simulink model "Simulation"  (R2020b)
settings: Solver=VariableStepAuto  StartTime=0.0  StopTime=10  RelTol=1e-3
model workspace (MAT data in the model file):
  DGain = Simulink.Parameter
  DGain.DataType = 'auto'
  DGain.Dimensions = [0 0]
  IGain = Simulink.Parameter
  IGain.DataType = 'auto'
  IGain.Dimensions = [0 0]
  PGain = Simulink.Parameter
  PGain.DataType = 'auto'
  PGain.Dimensions = [0 0]
libraries: aerolibconvert2 x2, shared3dof x1
settings Model: Creator=salaa  LastModifiedBy=salaa

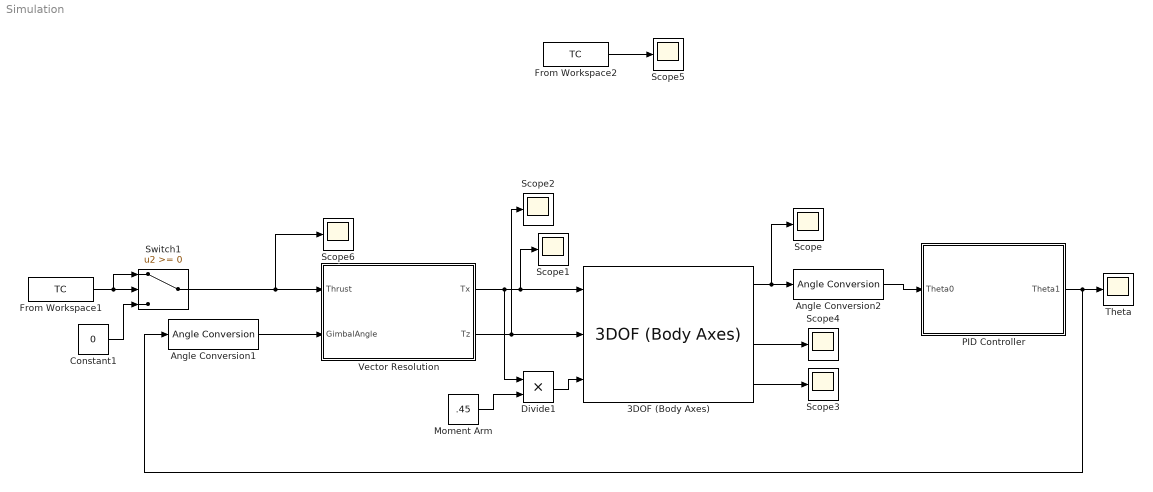
== system Simulation ==
  3DOF (Body Axes) : shared3dof/3DOF (Body Axes)  units=Metric (MKS)  mtype=Fixed  v_ini=0  theta_ini=0.01  alpha_ini=0  pos_ini=[0 0]  q_ini=0  mass=0.68  mass_e=0.5  mass_f=3.0  Iyy=1.0  Iyy_e=0.5  Iyy_f=3.0  g_in=Internal  g=-9.81  vre_flag=on  abi_flag=off  aMode=0  vel_statename=''  theta_statename=''  pos_statename=''  q_statename=''  mass_statename=''
      settings: SourceProductBaseCode=AE,PW,MT,UV,VE,VP
  Angle Conversion1 : aerolibconvert2/Angle Conversion  IU=deg  OU=rad
  Angle Conversion2 : aerolibconvert2/Angle Conversion  IU=rad  OU=deg
  Constant1 : Constant  Value=0
  Divide1 : Product  Inputs=**
  From Workspace1 : FromWorkspace  VariableName=TC
  From Workspace2 : FromWorkspace  VariableName=TC
  "Moment Arm " : Constant  Value=.45
  PID Controller : Subsystem
  Scope{,1..6} (7 alike) : Scope
  Switch1 : Switch
  Theta : Scope
  Vector Resolution : Subsystem
  wires:
  From Workspace2/1 -> Scope5/1
  3DOF (Body Axes)/1 -> Scope/1, Angle Conversion2/1
  Angle Conversion1/1 -> Vector Resolution/2(GimbalAngle)
  Vector Resolution/1(Tx) -> Divide1/1, Scope1/1, 3DOF (Body Axes)/1
  Vector Resolution/2(Tz) -> Scope2/1, 3DOF (Body Axes)/2
  Divide1/1 -> 3DOF (Body Axes)/3
  "Moment Arm "/1 -> Divide1/2
  3DOF (Body Axes)/4 -> Scope4/1
  Angle Conversion2/1 -> PID Controller/1(Theta0)
  PID Controller/1(Theta1) -> Theta/1, Angle Conversion1/1
  From Workspace1/1 -> Switch1/1, Switch1/2
  Constant1/1 -> Switch1/3
  Switch1/1 -> Scope6/1, Vector Resolution/1(Thrust)
  3DOF (Body Axes)/6 -> Scope3/1

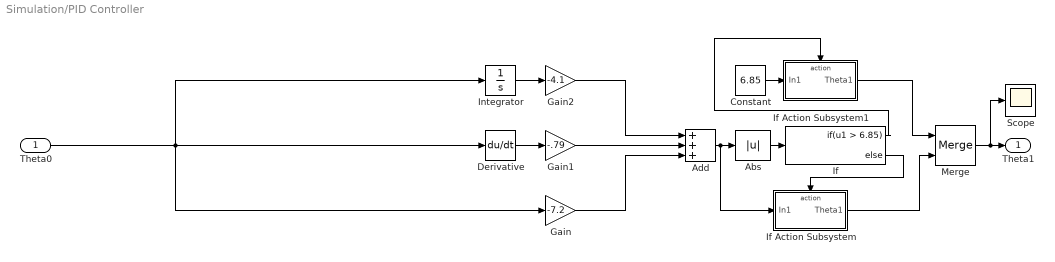
== system Simulation/PID Controller ==
  Theta0 : Inport
  Abs : Abs
  Add : Sum  Inputs=+++
  Constant : Constant  Value=6.85
  Derivative : Derivative
  Gain : Gain  Gain=-7.2
  Gain1 : Gain  Gain=-.79
  Gain2 : Gain  Gain=-4.1
  If : If  IfExpression=u1 > 6.85
  If Action Subsystem : Subsystem  TreatAsAtomicUnit=on
  If Action Subsystem1 : Subsystem  TreatAsAtomicUnit=on
  Integrator : Integrator
  Merge : Merge
  Scope : Scope
  Theta1 : Outport
  wires:
  Theta0/1 -> Integrator/1, Gain/1, Derivative/1
  Gain1/1 -> Add/2
  Gain/1 -> Add/3
  Derivative/1 -> Gain1/1
  Integrator/1 -> Gain2/1
  Gain2/1 -> Add/1
  Add/1 -> If Action Subsystem/1(In1), Abs/1
  Abs/1 -> If/1
  If/2 -> If Action Subsystem/Action
  If/1 -> If Action Subsystem1/Action
  Constant/1 -> If Action Subsystem1/1(In1)
  Merge/1 -> Scope/1, Theta1/1
  If Action Subsystem1/1(Theta1) -> Merge/1
  If Action Subsystem/1(Theta1) -> Merge/2

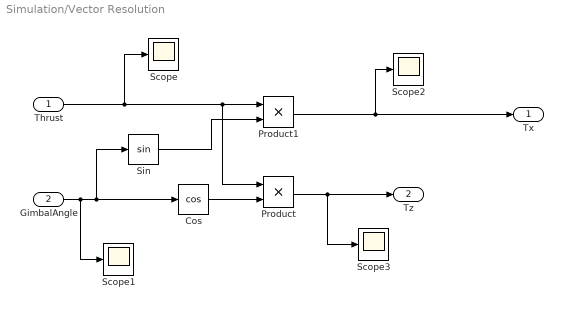
== system Simulation/Vector Resolution ==
  Thrust : Inport
  GimbalAngle : Inport  Port=2
  Cos : Trigonometry  Operator=cos
  Product : Product  RndMeth=Zero
  Product1 : Product  RndMeth=Zero
  Scope{,1..3} (4 alike) : Scope
  Sin : Trigonometry
  Tx : Outport
  Tz : Outport  Port=2
  wires:
  Product1/1 -> Scope2/1, Tx/1
  Cos/1 -> Product/2
  Product/1 -> Scope3/1, Tz/1
  Sin/1 -> Product1/2
  Thrust/1 -> Scope/1, Product/1, Product1/1
  GimbalAngle/1 -> Scope1/1, Cos/1, Sin/1

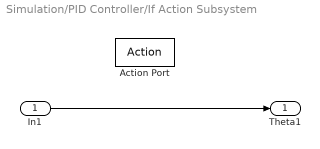
== system Simulation/PID Controller/If Action Subsystem ==
  In1 : Inport
  Action Port : ActionPort  ActionPortLabel=else
  Theta1 : Outport
  wires:
  In1/1 -> Theta1/1

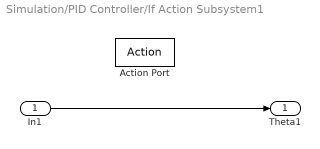
== system Simulation/PID Controller/If Action Subsystem1 ==
  In1 : Inport
  Action Port : ActionPort  ActionPortLabel=if(u1 > 6.85)
  Theta1 : Outport
  wires:
  In1/1 -> Theta1/1
